simulink model "cx06_MA"  (Simulink 7.5)
settings: Solver=FixedStepDiscrete  StartTime=0.0  StopTime=10.0  RelTol=1e-3
undefined symbols (not defined in the file or in its folder): DiscIntNeverNeededParam, ECU555, int, motohawk_build_version, motohawk_trunc_name, motohawk_vardec_path
libraries: MotoHawk_lib x811, simulink x43, simulink_need_slupdate x1
(part 5 of 10)

== system cx06_MA/Strategy/A/C Control Code ==
  In1 : Inport  OutDataType=sfix(16)  OutScaling=2^0
  A/C StateMachine : Stateflow chart  TreatAsAtomicUnit=on
  Bus Creator : BusCreator  Inputs=1
  Bus Selector : BusSelector  OutputSignals="GMLAN.AC_Clutch_Req,Analog.AC_Pres,Fiat.Engine  General Status.Eng_Running_Stat"
  Constant : Constant  OutDataType=sfix(16)  OutScaling=2^0
  Constant1 : Constant  Value=0  OutDataType=sfix(16)  OutScaling=2^0
  Logical Operator : Logic  Inputs=5  AllPortsSameDT=off  OutDataTypeMode=boolean  OutDataTypeStr=boolean
  Logical Operator1 : Logic  Operator=NOT  AllPortsSameDT=off  OutDataTypeMode=boolean  OutDataTypeStr=boolean
  Relational Operator : RelationalOperator  Operator===  LogicOutDataTypeMode=boolean  OutDataTypeStr=boolean
  Relational Operator1 : RelationalOperator  Operator=>  LogicOutDataTypeMode=boolean  OutDataTypeStr=boolean
  motohawk_calibration2 : MotoHawk_lib/Calibration & Probing Blocks/motohawk_calibration  nam='off_Pres'  val=10  storage=Calibration  show_more=on  name_source=Use Parameter  data_type=double  read_level=1  write_level=1  ovr_cals=on  view_as=Number  enum_struct={'False', 'True'}  vector_style=Wide Row  use_help_units=off  help=''  units=''  use_header_enum=off  row_header_enum={}  col_header_enum={}  use_min_max=on  min_val=0  max_val=inf  use_precision=on  precision='1.2'  gain=1  offset=0  exp=1  use_mototune_group=off  mototune_group=motohawk_vardec_path(gcb)
  motohawk_calibration3 : MotoHawk_lib/Calibration & Probing Blocks/motohawk_calibration  nam='on_Pres'  val=10  storage=Calibration  show_more=on  name_source=Use Parameter  data_type=double  read_level=1  write_level=1  ovr_cals=on  view_as=Number  enum_struct={'False', 'True'}  vector_style=Wide Row  use_help_units=off  help=''  units=''  use_header_enum=off  row_header_enum={}  col_header_enum={}  use_min_max=on  min_val=0  max_val=inf  use_precision=on  precision='1.2'  gain=1  offset=0  exp=1  use_mototune_group=off  mototune_group=motohawk_vardec_path(gcb)
  motohawk_calibration4 : MotoHawk_lib/Calibration & Probing Blocks/motohawk_calibration  nam='Enable_AC'  val=0  storage=Calibration  show_more=on  name_source=Use Parameter  data_type=uint16  read_level=1  write_level=1  ovr_cals=on  view_as=Enumeration  enum_struct={'False', 'True'}  vector_style=Wide Row  use_help_units=off  help=''  units=''  use_header_enum=off  row_header_enum={}  col_header_enum={}  use_min_max=on  min_val=-inf  max_val=inf  use_precision=on  precision=''  gain=1  offset=0  exp=1  use_mototune_group=off  mototune_group=motohawk_vardec_path(gcb)
  motohawk_fault_action : MotoHawk_lib/Fault Management Blocks/motohawk_fault_action  nam='inhibitAC'  output_status=on  eval_nam=inhibitAC
  motohawk_probe1 : MotoHawk_lib/Calibration & Probing Blocks/motohawk_probe  nam='HVAC_Req'  show_more=on  name_source=Use Parameter  read_level=1  view_as=Number  enum_struct={'Safety', 'Diesel', 'Regen', 'HEV', 'ZEV'}  vector_style=Wide Row  use_help_units=off  help=''  units=''  use_header_enum=off  row_header_enum={}  col_header_enum={}  use_precision=off  precision=''  gain=1  offset=0  exp=1  use_mototune_group=off  mototune_group=motohawk_vardec_path(gcb)
  motohawk_probe2 : MotoHawk_lib/Calibration & Probing Blocks/motohawk_probe  nam='AC_Pressure'  show_more=on  name_source=Use Parameter  read_level=1  view_as=Number  enum_struct={'Safety', 'Diesel', 'Regen', 'HEV', 'ZEV'}  vector_style=Wide Row  use_help_units=off  help=''  units=''  use_header_enum=off  row_header_enum={}  col_header_enum={}  use_precision=off  precision=''  gain=1  offset=0  exp=1  use_mototune_group=off  mototune_group=motohawk_vardec_path(gcb)
  motohawk_probe3 : MotoHawk_lib/Calibration & Probing Blocks/motohawk_probe  nam='Pres_In_Range'  show_more=on  name_source=Use Parameter  read_level=1  view_as=Number  enum_struct={'Safety', 'Diesel', 'Regen', 'HEV', 'ZEV'}  vector_style=Wide Row  use_help_units=off  help=''  units=''  use_header_enum=off  row_header_enum={}  col_header_enum={}  use_precision=off  precision=''  gain=1  offset=0  exp=1  use_mototune_group=off  mototune_group=motohawk_vardec_path(gcb)
  Out1 : Outport  OutDataType=sfix(16)  OutScaling=2^0
  wires:
  Bus Creator/1 -> Out1/1
  In1/1 -> Bus Selector/1
  Bus Selector/1 -> Relational Operator/2  "<AC_Clutch_Req>"
  Logical Operator/1 -> Bus Creator/1  "AC_On"
  Bus Selector/2 -> A/C StateMachine/1(Pressure), motohawk_probe2/1  "<AC_Pres>"
  motohawk_calibration2/1 -> A/C StateMachine/2(off_Pres)
  motohawk_calibration3/1 -> A/C StateMachine/3(on_Pres)
  A/C StateMachine/1(activate) -> motohawk_probe3/1, Logical Operator/5
  motohawk_calibration4/1 -> Logical Operator/1
  motohawk_fault_action/1 -> Logical Operator1/1
  Logical Operator1/1 -> Logical Operator/3
  Relational Operator/1 -> Logical Operator/2, motohawk_probe1/1
  Constant/1 -> Relational Operator/1
  Bus Selector/3 -> Relational Operator1/1  "<Eng_Running_Stat>"
  Constant1/1 -> Relational Operator1/2
  Relational Operator1/1 -> Logical Operator/4

== system cx06_MA/Strategy/Fiat/GMLAN Control Code ==
  In1 : Inport  OutDataType=sfix(16)  OutScaling=2^0
  Bus Creator : BusCreator  Inputs=1
  Gear Calc : Subsystem
  Gear_Estimation : Subsystem
  Neutral Check : Subsystem
  motohawk_probe : MotoHawk_lib/Calibration & Probing Blocks/motohawk_probe  nam='Estimated_Gear'  show_more=on  name_source=Use Parameter  read_level=1  view_as=Number  enum_struct={'Disabled', 'Enabled'}  vector_style=Wide Row  use_help_units=off  help=''  units=''  use_header_enum=off  row_header_enum={}  col_header_enum={}  use_precision=off  precision=''  gain=1  offset=0  exp=1  use_mototune_group=off  mototune_group=motohawk_vardec_path(gcb)
  motohawk_probe1 : MotoHawk_lib/Calibration & Probing Blocks/motohawk_probe  nam='Exp_Neutral_Fault'  show_more=on  name_source=Use Parameter  read_level=1  view_as=Number  enum_struct={'Disabled', 'Enabled'}  vector_style=Wide Row  use_help_units=off  help=''  units=''  use_header_enum=off  row_header_enum={}  col_header_enum={}  use_precision=off  precision=''  gain=1  offset=0  exp=1  use_mototune_group=off  mototune_group=motohawk_vardec_path(gcb)
  Out1 : Outport  OutDataType=sfix(16)  OutScaling=2^0
  wires:
  In1/1 -> Gear Calc/1(In1), Gear_Estimation/1(In1), Neutral Check/2(In1)
  Gear Calc/1(gear) -> Bus Creator/1  "gear"
  Bus Creator/1 -> Out1/1
  Gear_Estimation/1(gear) -> Neutral Check/1(gear_In), Gear Calc/2(gear_In), motohawk_probe/1
  Neutral Check/1(fault) -> motohawk_probe1/1

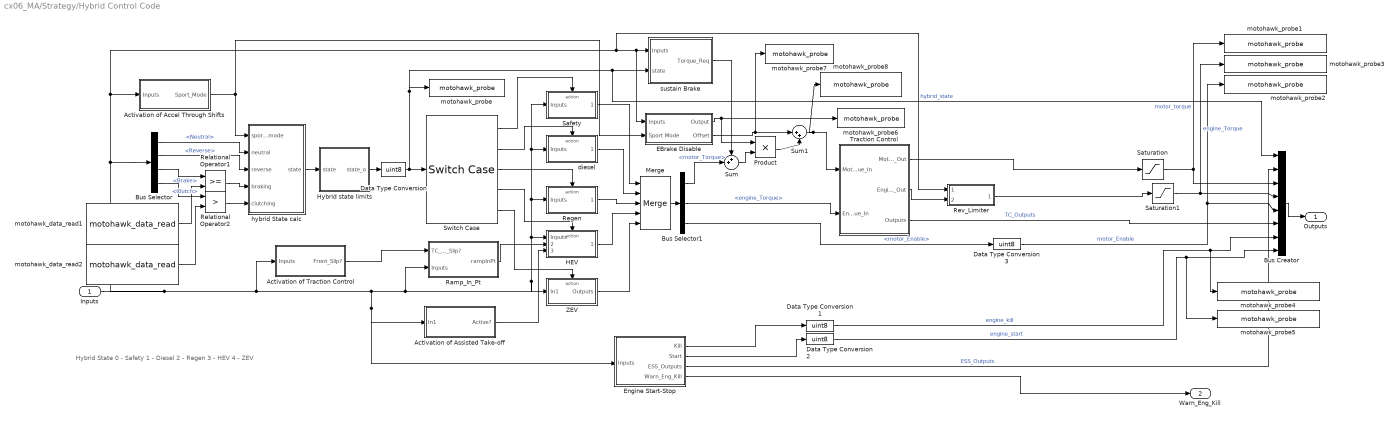
== system cx06_MA/Strategy/Hybrid Control Code ==
  note: Hybrid State
      | 0 - Safety
      | 1 - Diesel
      | 2 - Regen
      | 3 - HEV
      | 4 - ZEV
  Inputs : Inport  OutDataType=sfix(16)  OutScaling=2^0
  Activation of Accel Through Shifts : Subsystem
  Activation of Assisted Take-off : Subsystem
  Activation of Traction Control : Subsystem
  Bus Creator : BusCreator  Inputs=8
  Bus Selector : BusSelector  OutputSignals=Analog.Trans.Neutral,Analog.Trans.Reverse,Analog.Driver.Brake,Analog.Driver.Clutch
  Bus Selector1 : BusSelector  OutputSignals=motor_Torque,engine_Torque,motor_Enable
  Data Type Conversion{,1..3} (4 alike) : DataTypeConversion  OutDataTypeMode=uint8  OutDataType=sfix(16)  OutScaling=2^0  OutDataTypeStr=uint8
  EBrake Disable : Subsystem
  Engine Start-Stop : Subsystem
  HEV : Subsystem  TreatAsAtomicUnit=on
  Hybrid state limits : Subsystem
  Merge : Merge  Inputs=5
  Product : Product  OutDataType=sfix(16)  OutScaling=2^0  RndMeth=Zero
  Ramp_In_Pt : Subsystem
  Regen : Subsystem  TreatAsAtomicUnit=on
  Relational Operator1 : RelationalOperator  LogicOutDataTypeMode=boolean  OutDataTypeStr=boolean
  Relational Operator2 : RelationalOperator  Operator=>  LogicOutDataTypeMode=boolean  OutDataTypeStr=boolean
  Rev_Limiter : Subsystem
  Safety : Subsystem  TreatAsAtomicUnit=on
  Saturation : Saturate  UpperLimit=1  LowerLimit=-1
  Saturation1 : Saturate  UpperLimit=1  LowerLimit=0
  Sum : Sum  Inputs=++|  OutDataType=sfix(16)  OutScaling=2^0
  Sum1 : Sum  Inputs=|++  OutDataType=sfix(16)  OutScaling=2^0
  Switch Case : SwitchCase  CaseConditions={0,1,2,3,4}  ShowDefaultCase=off
  Traction Control : Subsystem
  ZEV : Subsystem  TreatAsAtomicUnit=on
  diesel : Subsystem  TreatAsAtomicUnit=on
  hybrid State calc : Stateflow chart  TreatAsAtomicUnit=on
  motohawk_data_read1 : MotoHawk_lib/Data Storage Blocks/motohawk_data_read  source=Lookup By Name  structure=Scalar  operation=Read scalar from location by index  sz_vec=4  sz_row=2  sz_col=3  typ=double  nam='Regen_Start'  checkNull=on  struct_inst_name='Struct1'  struct_nam='MyStruct'
  motohawk_data_read2 : MotoHawk_lib/Data Storage Blocks/motohawk_data_read  source=Lookup By Name  structure=Scalar  operation=Read scalar from location by index  sz_vec=4  sz_row=2  sz_col=3  typ=double  nam='AT_Start'  checkNull=on  struct_inst_name='Struct1'  struct_nam='MyStruct'
  motohawk_probe : MotoHawk_lib/Calibration & Probing Blocks/motohawk_probe  nam='Hybrid_State'  show_more=on  name_source=Use Parameter  read_level=1  view_as=Enumeration  enum_struct={'Safety', 'Diesel', 'Regen', 'HEV', 'ZEV'}  vector_style=Wide Row  use_help_units=off  help=''  units=''  use_header_enum=off  row_header_enum={}  col_header_enum={}  use_precision=off  precision=''  gain=1  offset=0  exp=1  use_mototune_group=off  mototune_group=motohawk_vardec_path(gcb)
  motohawk_probe1 : MotoHawk_lib/Calibration & Probing Blocks/motohawk_probe  nam='motor_Torque'  show_more=on  name_source=Use Parameter  read_level=1  view_as=Number  enum_struct={'Disabled', 'Enabled'}  vector_style=Wide Row  use_help_units=off  help=''  units=''  use_header_enum=off  row_header_enum={}  col_header_enum={}  use_precision=on  precision='1.3'  gain=1  offset=0  exp=1  use_mototune_group=off  mototune_group=motohawk_vardec_path(gcb)
  motohawk_probe2 : MotoHawk_lib/Calibration & Probing Blocks/motohawk_probe  nam='motor_Enable'  show_more=on  name_source=Use Parameter  read_level=1  view_as=Enumeration  enum_struct={'FALSE', 'true'}  vector_style=Wide Row  use_help_units=off  help=''  units=''  use_header_enum=off  row_header_enum={}  col_header_enum={}  use_precision=off  precision=''  gain=1  offset=0  exp=1  use_mototune_group=off  mototune_group=motohawk_vardec_path(gcb)
  motohawk_probe3 : MotoHawk_lib/Calibration & Probing Blocks/motohawk_probe  nam='diesel_Torque'  show_more=on  name_source=Use Parameter  read_level=1  view_as=Number  enum_struct={'Disabled', 'Enabled'}  vector_style=Wide Row  use_help_units=off  help=''  units=''  use_header_enum=off  row_header_enum={}  col_header_enum={}  use_precision=on  precision='1.3'  gain=1  offset=0  exp=1  use_mototune_group=off  mototune_group=motohawk_vardec_path(gcb)
  motohawk_probe4 : MotoHawk_lib/Calibration & Probing Blocks/motohawk_probe  nam='eng_Kill'  show_more=on  name_source=Use Parameter  read_level=1  view_as=Enumeration  enum_struct={'False', 'True'}  vector_style=Wide Row  use_help_units=off  help=''  units=''  use_header_enum=off  row_header_enum={}  col_header_enum={}  use_precision=on  precision=''  gain=1  offset=0  exp=1  use_mototune_group=off  mototune_group=motohawk_vardec_path(gcb)
  motohawk_probe5 : MotoHawk_lib/Calibration & Probing Blocks/motohawk_probe  nam='eng_Start'  show_more=on  name_source=Use Parameter  read_level=1  view_as=Enumeration  enum_struct={'False', 'True'}  vector_style=Wide Row  use_help_units=off  help=''  units=''  use_header_enum=off  row_header_enum={}  col_header_enum={}  use_precision=on  precision=''  gain=1  offset=0  exp=1  use_mototune_group=off  mototune_group=motohawk_vardec_path(gcb)
  motohawk_probe6 : MotoHawk_lib/Calibration & Probing Blocks/motohawk_probe  nam='EBrake_Multiplier'  show_more=on  name_source=Use Parameter  read_level=1  view_as=Number  enum_struct={'False', 'True'}  vector_style=Wide Row  use_help_units=off  help=''  units=''  use_header_enum=off  row_header_enum={}  col_header_enum={}  use_precision=on  precision='1.1'  gain=1  offset=0  exp=1  use_mototune_group=off  mototune_group=motohawk_vardec_path(gcb)
  motohawk_probe7 : MotoHawk_lib/Calibration & Probing Blocks/motohawk_probe  nam='EBrake_Offset'  show_more=on  name_source=Use Parameter  read_level=1  view_as=Number  enum_struct={'False', 'True'}  vector_style=Wide Row  use_help_units=off  help=''  units=''  use_header_enum=off  row_header_enum={}  col_header_enum={}  use_precision=on  precision='1.3'  gain=1  offset=0  exp=1  use_mototune_group=off  mototune_group=motohawk_vardec_path(gcb)
  motohawk_probe8 : MotoHawk_lib/Calibration & Probing Blocks/motohawk_probe  nam='Motor_Torque_Pre_Filt'  show_more=on  name_source=Use Parameter  read_level=1  view_as=Number  enum_struct={'False', 'True'}  vector_style=Wide Row  use_help_units=off  help=''  units=''  use_header_enum=off  row_header_enum={}  col_header_enum={}  use_precision=on  precision='1.3'  gain=1  offset=0  exp=1  use_mototune_group=off  mototune_group=motohawk_vardec_path(gcb)
  sustain Brake : Subsystem
  Outputs : Outport  OutDataType=sfix(16)  OutScaling=2^0
  Warn_Eng_Kill : Outport  Port=2  OutDataType=sfix(16)  OutScaling=2^0
  wires:
  Inputs/1 -> Bus Selector/1, Activation of Accel Through Shifts/1(Inputs), sustain Brake/1(Inputs), EBrake Disable/1(Inputs), Rev_Limiter/1(Inputs), ZEV/1(In1), HEV/1(Inputs), Safety/1(Inputs), diesel/1(Inputs), Regen/1(Inputs), Ramp_In_Pt/2(Inputs), Activation of Assisted Take-off/1(In1), Engine Start-Stop/1(Inputs), Activation of Traction Control/1(Inputs)
  Safety/1(Outputs) -> Merge/1
  diesel/1(Outputs) -> Merge/2
  HEV/1(Outputs) -> Merge/4
  ZEV/1(Outputs) -> Merge/5
  Regen/1(Outputs) -> Merge/3
  Switch Case/3 -> Regen/Action
  Switch Case/4 -> HEV/Action
  Switch Case/5 -> ZEV/Action
  Switch Case/2 -> diesel/Action
  Switch Case/1 -> Safety/Action
  Hybrid state limits/1(state_o) -> Data Type Conversion/1
  hybrid State calc/1(state) -> Hybrid state limits/1(state)
  Bus Selector/1 -> hybrid State calc/2(neutral)  "<Neutral>"
  Bus Selector/2 -> hybrid State calc/3(reverse)  "<Reverse>"
  Bus Selector/3 -> Relational Operator1/1  "<Brake>"
  Bus Selector/4 -> Relational Operator2/1  "<Clutch>"
  Relational Operator1/1 -> hybrid State calc/4(braking)
  Relational Operator2/1 -> hybrid State calc/5(clutching)
  motohawk_data_read1/1 -> Relational Operator1/2
  motohawk_data_read2/1 -> Relational Operator2/2
  Merge/1 -> Bus Selector1/1
  sustain Brake/1(Torque_Req) -> Sum/1
  Bus Selector1/1 -> Sum/2  "<motor_Torque>"
  Bus Creator/1 -> Outputs/1
  Data Type Conversion/1 -> Switch Case/1, motohawk_probe/1, sustain Brake/2("state "), Bus Creator/1  "hybrid_state"
  Data Type Conversion1/1 -> motohawk_probe4/1, Bus Creator/7  "engine_kill"
  Data Type Conversion2/1 -> motohawk_probe5/1, Bus Creator/8  "engine_start"
  Ramp_In_Pt/1(rampInPt) -> HEV/2(RampInPt)
  Traction Control/2(Engine_Torque_Out) -> Rev_Limiter/2(Torq_In)
  Saturation1/1 -> motohawk_probe3/1, Bus Creator/4  "engine_Torque"
  Saturation/1 -> motohawk_probe1/1, Bus Creator/3  "motor_torque"
  Bus Selector1/2 -> Traction Control/2(Engine_Torque_In)  "<engine_Torque>"
  Bus Selector1/3 -> Data Type Conversion3/1  "<motor_Enable>"
  Data Type Conversion3/1 -> motohawk_probe2/1, Bus Creator/5  "motor_Enable"
  Activation of Assisted Take-off/1(Active?) -> HEV/3(Activate_AT?)
  Activation of Traction Control/1(Front_Slip?) -> Ramp_In_Pt/1(TC_Front_Slip?)
  Activation of Accel Through Shifts/1(Sport_Mode) -> hybrid State calc/1(sport_mode), EBrake Disable/2(Sport Mode)
  Engine Start-Stop/3(ESS_Outputs) -> Bus Creator/2  "ESS_Outputs"
  Engine Start-Stop/1(Kill) -> Data Type Conversion1/1
  Engine Start-Stop/2(Start) -> Data Type Conversion2/1
  Traction Control/1(Motor_Torque_Out) -> Saturation/1
  Traction Control/3(Outputs) -> Bus Creator/6  "TC_Outputs"
  Rev_Limiter/1(Torq_Out) -> Saturation1/1
  EBrake Disable/1(Output) -> Product/1, motohawk_probe6/1
  Engine Start-Stop/4(Warn_Eng_Kill) -> Warn_Eng_Kill/1
  Sum/1 -> Product/2
  EBrake Disable/2(Offset) -> Sum1/1, motohawk_probe7/1
  Product/1 -> Sum1/2
  Sum1/1 -> Traction Control/1(Motor_Torque_In), motohawk_probe8/1

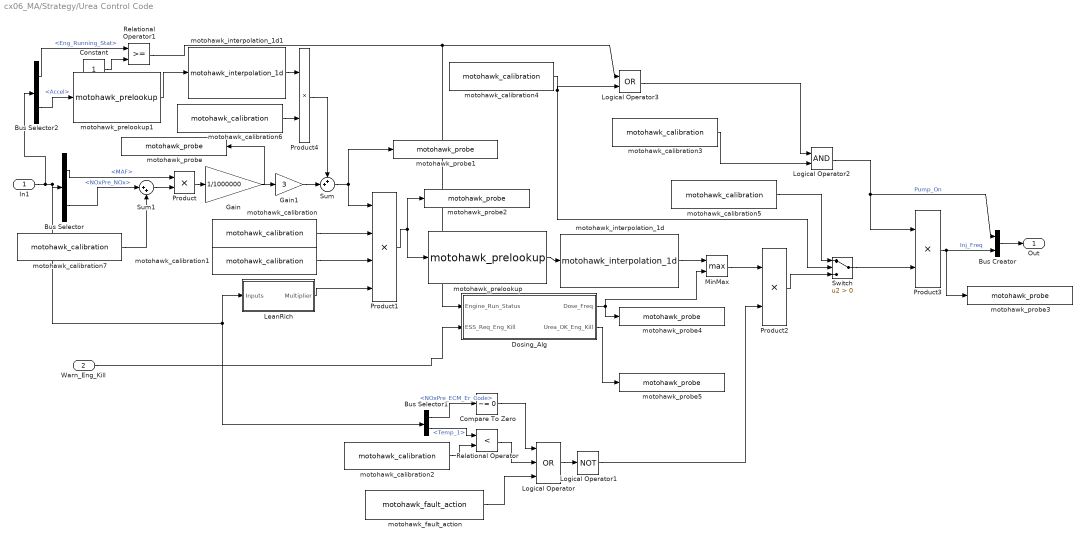
== system cx06_MA/Strategy/Urea Control Code ==
  In1 : Inport  OutDataType=sfix(16)  OutScaling=2^0
  Warn_Eng_Kill : Inport  Port=2  OutDataType=sfix(16)  OutScaling=2^0
  Bus Creator : BusCreator  Inputs=2
  Bus Selector : BusSelector  OutputSignals=Analog.MAF,Urea.NOx_Pre.NOxPre_NOx
  Bus Selector1 : BusSelector  OutputSignals=Urea.NOx_Pre.NOxPre_ECM_Er_Code,Urea.Temperature.Temp_1
  Bus Selector2 : BusSelector  OutputSignals="Fiat.Engine  General Status.Eng_Running_Stat,Analog.Driver.Accel"
  Compare To Zero : simulink/Logic and Bit Operations/Compare To Zero  SystemSampleTime=-1  relop=~=  LogicOutDataTypeMode=uint8  ZeroCross=off
  Constant : Constant  OutDataType=sfix(16)  OutScaling=2^0
  Dosing_Alg : Subsystem
  Gain : Gain  Gain=1/1000000  ParameterDataType=sfix(16)  ParameterScaling=2^0  OutDataType=sfix(16)  OutScaling=2^0
  Gain1 : Gain  Gain=3  ParameterDataType=sfix(16)  ParameterScaling=2^0  OutDataType=sfix(16)  OutScaling=2^0
  LeanRich : Subsystem
  Logical Operator : Logic  Operator=OR  Inputs=3  AllPortsSameDT=off  OutDataTypeMode=boolean  OutDataTypeStr=boolean
  Logical Operator1 : Logic  Operator=NOT  AllPortsSameDT=off  OutDataTypeMode=boolean  OutDataTypeStr=boolean
  Logical Operator2 : Logic  AllPortsSameDT=off  OutDataTypeMode=boolean  OutDataTypeStr=boolean
  Logical Operator3 : Logic  Operator=OR  AllPortsSameDT=off  OutDataTypeMode=boolean  OutDataTypeStr=boolean
  MinMax : MinMax  Function=max  Inputs=2  OutDataType=sfix(16)  OutScaling=2^0
  Product{,2..4} (4 alike) : Product  OutDataType=sfix(16)  OutScaling=2^0  RndMeth=Zero
  Product1 : Product  Inputs=4  OutDataType=sfix(16)  OutScaling=2^0  RndMeth=Zero
  Relational Operator : RelationalOperator  Operator=<  LogicOutDataTypeMode=boolean  OutDataTypeStr=boolean
  Relational Operator1 : RelationalOperator  LogicOutDataTypeMode=boolean  OutDataTypeStr=boolean
  Sum : Sum  Inputs=++|  OutDataType=sfix(16)  OutScaling=2^0
  Sum1 : Sum  Inputs=|++  OutDataType=sfix(16)  OutScaling=2^0
  Switch : Switch  Criteria=u2 > Threshold
  motohawk_calibration : MotoHawk_lib/Calibration & Probing Blocks/motohawk_calibration  nam='Urea_Dilution'  val=0  storage=Calibration  show_more=on  name_source=Use Parameter  data_type=Inherit from 'Default Value'  read_level=1  write_level=1  ovr_cals=on  view_as=Number  enum_struct={'Disabled', 'Enabled'}  vector_style=Wide Row  use_help_units=on  help='Dilution multiplier ureaMass * Urea_Dilution = SolutionMass'  units=''  use_header_enum=off  row_header_enum={}  col_header_enum={}  use_min_max=off  min_val=-inf  max_val=inf  use_precision=on  precision='1.3'  gain=1  offset=0  exp=1  use_mototune_group=off  mototune_group=motohawk_vardec_path(gcb)
  motohawk_calibration1 : MotoHawk_lib/Calibration & Probing Blocks/motohawk_calibration  nam='UreaNOx_Mult'  val=0  storage=Calibration  show_more=on  name_source=Use Parameter  data_type=Inherit from 'Default Value'  read_level=1  write_level=1  ovr_cals=on  view_as=Number  enum_struct={'Disabled', 'Enabled'}  vector_style=Wide Row  use_help_units=on  help='Multiplier to increase injection from NOx path'  units=''  use_header_enum=off  row_header_enum={}  col_header_enum={}  use_min_max=off  min_val=-inf  max_val=inf  use_precision=on  precision='1.3'  gain=1  offset=0  exp=1  use_mototune_group=off  mototune_group=motohawk_vardec_path(gcb)
  motohawk_calibration2 : MotoHawk_lib/Calibration & Probing Blocks/motohawk_calibration  nam='UreaMin_Temp'  val=0  storage=Calibration  show_more=on  name_source=Use Parameter  data_type=Inherit from 'Default Value'  read_level=1  write_level=1  ovr_cals=on  view_as=Number  enum_struct={'Disabled', 'Enabled'}  vector_style=Wide Row  use_help_units=on  help='Exhaust must be this hot to inject'  units=''  use_header_enum=off  row_header_enum={}  col_header_enum={}  use_min_max=off  min_val=-inf  max_val=inf  use_precision=on  precision='1.3'  gain=1  offset=0  exp=1  use_mototune_group=off  mototune_group=motohawk_vardec_path(gcb)
  motohawk_calibration3 : MotoHawk_lib/Calibration & Probing Blocks/motohawk_calibration  nam='Urea_Enable'  val=0  storage=Calibration  show_more=on  name_source=Use Parameter  data_type=boolean  read_level=1  write_level=1  ovr_cals=on  view_as=Enumeration  enum_struct={'Disabled', 'Enabled'}  vector_style=Wide Row  use_help_units=on  help=''  units=''  use_header_enum=off  row_header_enum={}  col_header_enum={}  use_min_max=off  min_val=-inf  max_val=inf  use_precision=on  precision='1.3'  gain=1  offset=0  exp=1  use_mototune_group=off  mototune_group=motohawk_vardec_path(gcb)
  motohawk_calibration4 : MotoHawk_lib/Calibration & Probing Blocks/motohawk_calibration  nam='Urea_Purge'  val=0  storage=Calibration  show_more=on  name_source=Use Parameter  data_type=boolean  read_level=1  write_level=1  ovr_cals=on  view_as=Enumeration  enum_struct={'Disabled', 'Enabled'}  vector_style=Wide Row  use_help_units=on  help='Set Injection to a fixed rate'  units=''  use_header_enum=off  row_header_enum={}  col_header_enum={}  use_min_max=off  min_val=-inf  max_val=inf  use_precision=on  precision='1.3'  gain=1  offset=0  exp=1  use_mototune_group=off  mototune_group=motohawk_vardec_path(gcb)
  motohawk_calibration5 : MotoHawk_lib/Calibration & Probing Blocks/motohawk_calibration  nam='Urea_PurgeLevel'  val=0  storage=Calibration  show_more=on  name_source=Use Parameter  data_type=Inherit from 'Default Value'  read_level=1  write_level=1  ovr_cals=on  view_as=Number  enum_struct={'Disabled', 'Enabled'}  vector_style=Wide Row  use_help_units=on  help=''  units='Hz'  use_header_enum=off  row_header_enum={}  col_header_enum={}  use_min_max=off  min_val=-inf  max_val=inf  use_precision=on  precision='1.1'  gain=1  offset=0  exp=1  use_mototune_group=off  mototune_group=motohawk_vardec_path(gcb)
  motohawk_calibration6 : MotoHawk_lib/Calibration & Probing Blocks/motohawk_calibration  nam='UreaAccel_Mult'  val=0  storage=Calibration  show_more=on  name_source=Use Parameter  data_type=Inherit from 'Default Value'  read_level=1  write_level=1  ovr_cals=on  view_as=Number  enum_struct={'Disabled', 'Enabled'}  vector_style=Wide Row  use_help_units=on  help='Multiplier to increase injection from NOx path'  units=''  use_header_enum=off  row_header_enum={}  col_header_enum={}  use_min_max=off  min_val=-inf  max_val=inf  use_precision=on  precision='1.3'  gain=1  offset=0  exp=1  use_mototune_group=off  mototune_group=motohawk_vardec_path(gcb)
  motohawk_calibration7 : MotoHawk_lib/Calibration & Probing Blocks/motohawk_calibration  nam='NOx_Offset'  val=0  storage=Calibration  show_more=on  name_source=Use Parameter  data_type=uint16  read_level=1  write_level=1  ovr_cals=on  view_as=Number  enum_struct={'Disabled', 'Enabled'}  vector_style=Wide Row  use_help_units=on  help='Dilution multiplier ureaMass * Urea_Dilution = SolutionMass'  units=''  use_header_enum=off  row_header_enum={}  col_header_enum={}  use_min_max=off  min_val=-inf  max_val=inf  use_precision=on  precision='1.1'  gain=1  offset=0  exp=1  use_mototune_group=off  mototune_group=motohawk_vardec_path(gcb)
  motohawk_fault_action : MotoHawk_lib/Fault Management Blocks/motohawk_fault_action  nam='Urea_Inject'  output_status=on  eval_nam=Urea_Inject
  motohawk_interpolation_1d : MotoHawk_lib/Lookup Tables/motohawk_interpolation_1d  nam='Urea_Injection_Tbl'  table_data=1:1:10  show_more=on  data_type=Inherit from 'Table Data'  storage=NonAdaptive  read_level=1  write_level=1  ovr_cals=on  use_help=off  help=''  units=''  use_min_max=off  min_val=-inf  max_val=inf  use_precision=off  precision=''  gain=1  offset=0  exp=1  use_links=on  prelookup_block='Urea_Injection_Ord'  output_name=''  use_mototune_group=off  mototune_group=motohawk_vardec_path(gcb)
  motohawk_interpolation_1d1 : MotoHawk_lib/Lookup Tables/motohawk_interpolation_1d  nam='Urea_Accel_Tbl'  table_data=1:1:10  show_more=on  data_type=Inherit from 'Table Data'  storage=NonAdaptive  read_level=1  write_level=1  ovr_cals=on  use_help=off  help=''  units=''  use_min_max=off  min_val=-inf  max_val=inf  use_precision=off  precision=''  gain=1  offset=0  exp=1  use_links=on  prelookup_block='Urea_Accel_Ord'  output_name=''  use_mototune_group=off  mototune_group=motohawk_vardec_path(gcb)
  motohawk_prelookup : MotoHawk_lib/Lookup Tables/motohawk_prelookup  nam='Urea_Injection_Ord'  breakpoint_data=1:1:10  show_more=off  data_type=Inherit from 'Table Data'  storage=Constant  read_level=1  write_level=1  ovr_cals=on  use_help=off  help=''  units=''  use_min_max=off  min_val=-inf  max_val=inf  use_precision=off  precision=''  gain=1  offset=0  exp=1  use_links=off  input_name=''  use_mototune_group=off  mototune_group=motohawk_vardec_path(gcb)
  motohawk_prelookup1 : MotoHawk_lib/Lookup Tables/motohawk_prelookup  nam='Urea_Accel_Ord'  breakpoint_data=1:1:10  show_more=off  data_type=Inherit from 'Table Data'  storage=Constant  read_level=1  write_level=1  ovr_cals=on  use_help=off  help=''  units=''  use_min_max=off  min_val=-inf  max_val=inf  use_precision=off  precision=''  gain=1  offset=0  exp=1  use_links=off  input_name=''  use_mototune_group=off  mototune_group=motohawk_vardec_path(gcb)
  motohawk_probe : MotoHawk_lib/Calibration & Probing Blocks/motohawk_probe  nam='NOx_MFlow_Theory'  show_more=on  name_source=Use Parameter  read_level=1  view_as=Number  enum_struct={'Disabled', 'Enabled'}  vector_style=Wide Row  use_help_units=off  help=''  units=''  use_header_enum=off  row_header_enum={}  col_header_enum={}  use_precision=on  precision='1.3'  gain=1  offset=0  exp=1  use_mototune_group=off  mototune_group=motohawk_vardec_path(gcb)
  motohawk_probe1 : MotoHawk_lib/Calibration & Probing Blocks/motohawk_probe  nam='Urea_MFlow'  show_more=on  name_source=Use Parameter  read_level=1  view_as=Number  enum_struct={'Disabled', 'Enabled'}  vector_style=Wide Row  use_help_units=off  help=''  units=''  use_header_enum=off  row_header_enum={}  col_header_enum={}  use_precision=on  precision='1.3'  gain=1  offset=0  exp=1  use_mototune_group=off  mototune_group=motohawk_vardec_path(gcb)
  motohawk_probe2 : MotoHawk_lib/Calibration & Probing Blocks/motohawk_probe  nam='Solution_MFlow'  show_more=on  name_source=Use Parameter  read_level=1  view_as=Number  enum_struct={'Disabled', 'Enabled'}  vector_style=Wide Row  use_help_units=off  help=''  units=''  use_header_enum=off  row_header_enum={}  col_header_enum={}  use_precision=on  precision='1.3'  gain=1  offset=0  exp=1  use_mototune_group=off  mototune_group=motohawk_vardec_path(gcb)
  motohawk_probe3 : MotoHawk_lib/Calibration & Probing Blocks/motohawk_probe  nam='UreaInj_Freq'  show_more=off  name_source=Use Parameter  read_level=1  view_as=Number  enum_struct={'Disabled', 'Enabled'}  vector_style=Wide Row  use_help_units=off  help=''  units=''  use_header_enum=off  row_header_enum={}  col_header_enum={}  use_precision=off  precision=''  gain=1  offset=0  exp=1  use_mototune_group=off  mototune_group=motohawk_vardec_path(gcb)
  motohawk_probe4 : MotoHawk_lib/Calibration & Probing Blocks/motohawk_probe  nam='Dosing_Freq'  show_more=on  name_source=Use Parameter  read_level=1  view_as=Number  enum_struct={'Disabled', 'Enabled'}  vector_style=Wide Row  use_help_units=off  help=''  units=''  use_header_enum=off  row_header_enum={}  col_header_enum={}  use_precision=on  precision='1.3'  gain=1  offset=0  exp=1  use_mototune_group=off  mototune_group=motohawk_vardec_path(gcb)
  motohawk_probe5 : MotoHawk_lib/Calibration & Probing Blocks/motohawk_probe  nam='Urea_OK_Eng_Kill'  show_more=on  name_source=Use Parameter  read_level=1  view_as=Number  enum_struct={'Disabled', 'Enabled'}  vector_style=Wide Row  use_help_units=off  help=''  units=''  use_header_enum=off  row_header_enum={}  col_header_enum={}  use_precision=on  precision='1.1'  gain=1  offset=0  exp=1  use_mototune_group=off  mototune_group=motohawk_vardec_path(gcb)
  Out : Outport  OutDataType=sfix(16)  OutScaling=2^0
  wires:
  In1/1 -> Bus Selector/1, Bus Selector1/1, LeanRich/1(Inputs), Bus Selector2/1
  Bus Selector/1 -> Product/1  "<MAF>"
  Product/1 -> Gain/1
  Gain/1 -> motohawk_probe/1, Gain1/1
  motohawk_calibration/1 -> Product1/2
  Product1/1 -> motohawk_probe2/1, motohawk_prelookup/1
  motohawk_calibration1/1 -> Product1/3
  motohawk_prelookup/1 -> motohawk_interpolation_1d/1
  Bus Selector1/2 -> Relational Operator/1  "<Temp_1>"
  motohawk_calibration2/1 -> Relational Operator/2
  Logical Operator/1 -> Logical Operator1/1
  Logical Operator1/1 -> Product2/2
  Product2/1 -> Switch/3
  motohawk_calibration4/1 -> Switch/2, Logical Operator3/2
  motohawk_calibration5/1 -> Switch/1
  Switch/1 -> Product3/2
  Product3/1 -> Bus Creator/2, motohawk_probe3/1  "Inj_Freq"
  Bus Creator/1 -> Out/1
  Bus Selector1/1 -> Compare To Zero/1  "<NOxPre_ECM_Er_Code>"
  Compare To Zero/1 -> Logical Operator/1
  Relational Operator/1 -> Logical Operator/2
  motohawk_fault_action/1 -> Logical Operator/3
  motohawk_prelookup1/1 -> motohawk_interpolation_1d1/1
  motohawk_interpolation_1d1/1 -> Product4/1
  motohawk_calibration6/1 -> Product4/2
  Product4/1 -> Sum/1
  Gain1/1 -> Sum/2
  Sum/1 -> Product1/1, motohawk_probe1/1
  LeanRich/1(Multiplier) -> Product1/4
  Bus Selector2/2 -> motohawk_prelookup1/1  "<Accel>"
  motohawk_calibration3/1 -> Logical Operator2/2
  Logical Operator2/1 -> Product3/1, Bus Creator/1  "Pump_On"
  Logical Operator3/1 -> Logical Operator2/1
  Bus Selector2/1 -> Relational Operator1/1  "<Eng_Running_Stat>"
  Relational Operator1/1 -> Logical Operator3/1, Dosing_Alg/1(Engine_Run_Status)
  Constant/1 -> Relational Operator1/2
  motohawk_interpolation_1d/1 -> MinMax/1
  Dosing_Alg/1(Dose_Freq) -> MinMax/2, motohawk_probe4/1
  MinMax/1 -> Product2/1
  Warn_Eng_Kill/1 -> Dosing_Alg/2(ESS_Req_Eng_Kill)
  Dosing_Alg/2(Urea_OK_Eng_Kill) -> motohawk_probe5/1
  Sum1/1 -> Product/2
  motohawk_calibration7/1 -> Sum1/2
  Bus Selector/2 -> Sum1/1  "<NOxPre_NOx>"

== system cx06_MA/Inputs/Analog Inputs/AC_Pres ==
  Compare To Zero : simulink/Logic and Bit Operations/Compare To Zero  SystemSampleTime=-1  relop=~=  LogicOutDataTypeMode=boolean  ZeroCross=off
  Relational Operator : RelationalOperator  Operator=<  LogicOutDataTypeMode=boolean  OutDataTypeStr=boolean
  motohawk_ain1 : MotoHawk_lib/Analog I//O Blocks/motohawk_ain  res_name=[]  text_resource=(None)  code_resource=NONE  val_resource=-1  target=ECU555-80  resource_enum_str=(None)=-1,ECUP=53,DRVP=54,XDRP=55,AN1M=56,AN2M=57,AN3M=58,AN4M=59,AN5M=60,AN6M=61,AN7M=62,AN8M=63,AN9M=64,AN10M=65,AN11M=66,AN12M=67,AN13M=68,AN14M=69,AN15M=70,AN16M=71,AN17M=72,AN18M=73,AN19M=74,O2A=90,O2B=91,XDRP_B=92  altref=5V Reference  typ=uint16  num_adc_bits=10  use_stat=on  use_vardec=on  nam='AC_Pres'  read_level=1  write_level=1  group='I/O Pins | Inputs Config'
  motohawk_calibration1 : MotoHawk_lib/Calibration & Probing Blocks/motohawk_calibration  nam='min_Press_Thres'  val=10  storage=Calibration  show_more=on  name_source=Use Parameter  data_type=uint16  read_level=1  write_level=1  ovr_cals=on  view_as=Number  enum_struct={'False', 'True'}  vector_style=Wide Row  use_help_units=off  help=''  units=''  use_header_enum=off  row_header_enum={}  col_header_enum={}  use_min_max=on  min_val=-inf  max_val=inf  use_precision=on  precision=''  gain=1  offset=0  exp=1  use_mototune_group=off  mototune_group=motohawk_vardec_path(gcb)
  motohawk_fault_def1 : MotoHawk_lib/Fault Management Blocks/motohawk_fault_def  nam='ACAnalogErr'  mode=Enabled - Persistent  id=[]  x=10  y=20  input_suspected=on  indeterminate=off  increment_xy=on  downsample_count=1  ovr_cals=on  ovr_actions=on  show_actions=on  action1_name='inhibitAC'  action1_cond=Active  action2_name=''  action2_cond=(None)  action3_name=''  action3_cond=(None)  action4_name=''  action4_cond=(None)
  motohawk_fault_def3 : MotoHawk_lib/Fault Management Blocks/motohawk_fault_def  nam='ACLowPres'  mode=Enabled - Persistent  id=[]  x=10  y=20  input_suspected=on  indeterminate=off  increment_xy=on  downsample_count=1  ovr_cals=on  ovr_actions=on  show_actions=on  action1_name='inhibitAC'  action1_cond=Active  action2_name=''  action2_cond=(None)  action3_name=''  action3_cond=(None)  action4_name=''  action4_cond=(None)
  motohawk_interpolation_1d : MotoHawk_lib/Lookup Tables/motohawk_interpolation_1d  nam='AC_Cal_Tbl'  table_data=[1:1:9]  show_more=off  data_type=Inherit from 'Table Data'  storage=NonAdaptive  read_level=1  write_level=1  ovr_cals=on  use_help=off  help=''  units=''  use_min_max=off  min_val=-inf  max_val=inf  use_precision=off  precision=''  gain=1  offset=0  exp=1  use_links=off  prelookup_block=''  output_name=''  use_mototune_group=off  mototune_group=motohawk_vardec_path(gcb)
  motohawk_prelookup : MotoHawk_lib/Lookup Tables/motohawk_prelookup  nam='AC_Cal_Ord'  breakpoint_data=[0:128:1024]  show_more=on  data_type=uint16  storage=Constant  read_level=1  write_level=1  ovr_cals=off  use_help=off  help=''  units=''  use_min_max=off  min_val=-inf  max_val=inf  use_precision=off  precision=''  gain=1  offset=0  exp=1  use_links=off  input_name=''  use_mototune_group=off  mototune_group=motohawk_vardec_path(gcb)
  motohawk_probe1 : MotoHawk_lib/Calibration & Probing Blocks/motohawk_probe  nam='In_ACPres'  show_more=on  name_source=Use Parameter  read_level=1  view_as=Number  enum_struct={'Disabled', 'Enabled'}  vector_style=Wide Row  use_help_units=off  help=''  units=''  use_header_enum=off  row_header_enum={}  col_header_enum={}  use_precision=off  precision=''  gain=1  offset=0  exp=1  use_mototune_group=on  mototune_group='Debug | Inputs'
  AC_Pres : Outport  OutDataType=sfix(16)  OutScaling=2^0
  wires:
  motohawk_ain1/1 -> motohawk_prelookup/1
  motohawk_prelookup/1 -> motohawk_interpolation_1d/1
  motohawk_interpolation_1d/1 -> AC_Pres/1, Relational Operator/1  "AC_Pres"
  motohawk_ain1/2 -> motohawk_probe1/1, Compare To Zero/1
  motohawk_calibration1/1 -> Relational Operator/2
  Relational Operator/1 -> motohawk_fault_def3/1
  Compare To Zero/1 -> motohawk_fault_def1/1

== system cx06_MA/Inputs/Analog Inputs/Cruise Buttons ==
  note: 0 - (none)
      | 1 - on
      | 2 - on & up
      | 3 - on & down
  motohawk_ain2 : MotoHawk_lib/Analog I//O Blocks/motohawk_ain  res_name=[]  text_resource=AN5M  code_resource=NONE  val_resource=-1  target=ECU555-80  resource_enum_str=(None)=-1,ECUP=53,DRVP=54,XDRP=55,AN1M=56,AN2M=57,AN3M=58,AN4M=59,AN5M=60,AN6M=61,AN7M=62,AN8M=63,AN9M=64,AN10M=65,AN11M=66,AN12M=67,AN13M=68,AN14M=69,AN15M=70,AN16M=71,AN17M=72,AN18M=73,AN19M=74,O2A=90,O2B=91,XDRP_B=92  altref=5V Reference  typ=uint16  num_adc_bits=10  use_stat=on  use_vardec=on  nam='CruiseButtons'  read_level=1  write_level=1  group='I/O Pins | Inputs Config'
  motohawk_calibration1 : MotoHawk_lib/Calibration & Probing Blocks/motohawk_calibration  nam='Cruise_Main_Tres'  val=50  storage=Calibration  show_more=on  name_source=Use Parameter  data_type=Inherit via back propagation  read_level=1  write_level=1  ovr_cals=on  view_as=Number  enum_struct={'Disabled', 'Enabled'}  vector_style=Wide Row  use_help_units=off  help=''  units=''  use_header_enum=off  row_header_enum={}  col_header_enum={}  use_min_max=on  min_val=0  max_val=inf  use_precision=off  precision=''  gain=1  offset=0  exp=1  use_mototune_group=off  mototune_group=motohawk_vardec_path(gcb)
  motohawk_calibration2 : MotoHawk_lib/Calibration & Probing Blocks/motohawk_calibration  nam='Cruise_Up_Tres'  val=50  storage=Calibration  show_more=on  name_source=Use Parameter  data_type=Inherit via back propagation  read_level=1  write_level=1  ovr_cals=on  view_as=Number  enum_struct={'Disabled', 'Enabled'}  vector_style=Wide Row  use_help_units=off  help=''  units=''  use_header_enum=off  row_header_enum={}  col_header_enum={}  use_min_max=on  min_val=0  max_val=inf  use_precision=off  precision=''  gain=1  offset=0  exp=1  use_mototune_group=off  mototune_group=motohawk_vardec_path(gcb)
  motohawk_calibration3 : MotoHawk_lib/Calibration & Probing Blocks/motohawk_calibration  nam='Cruise_Down_Tres'  val=50  storage=Calibration  show_more=on  name_source=Use Parameter  data_type=Inherit via back propagation  read_level=1  write_level=1  ovr_cals=on  view_as=Number  enum_struct={'Disabled', 'Enabled'}  vector_style=Wide Row  use_help_units=off  help=''  units=''  use_header_enum=off  row_header_enum={}  col_header_enum={}  use_min_max=on  min_val=0  max_val=inf  use_precision=off  precision=''  gain=1  offset=0  exp=1  use_mototune_group=off  mototune_group=motohawk_vardec_path(gcb)
  motohawk_probe6 : MotoHawk_lib/Calibration & Probing Blocks/motohawk_probe  nam='In_CruiseButtons'  show_more=on  name_source=Use Parameter  read_level=1  view_as=Number  enum_struct={'Disabled', 'Enabled'}  vector_style=Wide Row  use_help_units=off  help=''  units=''  use_header_enum=off  row_header_enum={}  col_header_enum={}  use_precision=off  precision=''  gain=1  offset=0  exp=1  use_mototune_group=on  mototune_group='Debug | Inputs'
  motohawk_probe9 : MotoHawk_lib/Calibration & Probing Blocks/motohawk_probe  nam='raw_CruiseButton'  show_more=on  name_source=Use Parameter  read_level=1  view_as=Number  enum_struct={'Disabled', 'Enabled'}  vector_style=Wide Row  use_help_units=on  help=''  units=''  use_header_enum=off  row_header_enum={}  col_header_enum={}  use_precision=off  precision=''  gain=1  offset=0  exp=1  use_mototune_group=off  mototune_group=motohawk_vardec_path(gcb)
  read_Cruise_Buttons : Stateflow chart  TreatAsAtomicUnit=on
  Cruise_Button : Outport  OutDataType=sfix(16)  OutScaling=2^0
  wires:
  motohawk_ain2/2 -> motohawk_probe6/1
  motohawk_ain2/1 -> motohawk_probe9/1, read_Cruise_Buttons/1(u)
  motohawk_calibration1/1 -> read_Cruise_Buttons/2(b1)
  motohawk_calibration2/1 -> read_Cruise_Buttons/3(b2)
  motohawk_calibration3/1 -> read_Cruise_Buttons/4(b3)
  read_Cruise_Buttons/1(cruiseBut) -> Cruise_Button/1  "cruiseBut"

== system cx06_MA/Inputs/Analog Inputs/Driver Inputs ==
  Accel : Subsystem
  Brake : Subsystem
  Bus Creator : BusCreator  Inputs=3
  Clutch : Subsystem
  Driver : Outport  OutDataType=sfix(16)  OutScaling=2^0
  wires:
  Bus Creator/1 -> Driver/1
  Accel/1(Accel) -> Bus Creator/1  "Accel"
  Brake/1(Brake) -> Bus Creator/2  "Brake"
  Clutch/1(Clutch) -> Bus Creator/3  "Clutch"

== system cx06_MA/Inputs/Analog Inputs/Fuel Level ==
  2pt Calibration1_4 : Fcn  Expr=(u[1]-u[3])/(u[2]-u[3])
  Data Type Conversion3 : DataTypeConversion  OutDataTypeMode=single  OutDataType=sfix(16)  OutScaling=2^0  OutDataTypeStr=single
  Mux4 : Mux  Inputs=3
  Range_Detect : Subsystem
  Saturation3 : Saturate  UpperLimit=1  LowerLimit=0
  motohawk_ain3 : MotoHawk_lib/Analog I//O Blocks/motohawk_ain  res_name=[]  text_resource=AN13M  code_resource=NONE  val_resource=-1  target=ECU555-80  resource_enum_str=(None)=-1,ECUP=53,DRVP=54,XDRP=55,AN1M=56,AN2M=57,AN3M=58,AN4M=59,AN5M=60,AN6M=61,AN7M=62,AN8M=63,AN9M=64,AN10M=65,AN11M=66,AN12M=67,AN13M=68,AN14M=69,AN15M=70,AN16M=71,AN17M=72,AN18M=73,AN19M=74,O2A=90,O2B=91,XDRP_B=92  altref=5V Reference  typ=uint16  num_adc_bits=10  use_stat=on  use_vardec=on  nam='FuelLevel'  read_level=1  write_level=1  group='I/O Pins | Inputs Config'
  motohawk_calibration7 : MotoHawk_lib/Calibration & Probing Blocks/motohawk_calibration  nam='FeulLevel_Zero'  val=416  storage=Calibration  show_more=on  name_source=Use Parameter  data_type=Inherit via back propagation  read_level=1  write_level=1  ovr_cals=on  view_as=Number  enum_struct={'Disabled', 'Enabled'}  vector_style=Wide Row  use_help_units=off  help=''  units=''  use_header_enum=off  row_header_enum={}  col_header_enum={}  use_min_max=off  min_val=-inf  max_val=inf  use_precision=off  precision=''  gain=1  offset=0  exp=1  use_mototune_group=off  mototune_group=motohawk_vardec_path(gcb)
  motohawk_calibration8 : MotoHawk_lib/Calibration & Probing Blocks/motohawk_calibration  nam='FuelLevel_Full'  val=231  storage=Calibration  show_more=on  name_source=Use Parameter  data_type=Inherit via back propagation  read_level=1  write_level=1  ovr_cals=on  view_as=Number  enum_struct={'Disabled', 'Enabled'}  vector_style=Wide Row  use_help_units=off  help=''  units=''  use_header_enum=off  row_header_enum={}  col_header_enum={}  use_min_max=off  min_val=-inf  max_val=inf  use_precision=off  precision=''  gain=1  offset=0  exp=1  use_mototune_group=off  mototune_group=motohawk_vardec_path(gcb)
  motohawk_fault_def : MotoHawk_lib/Fault Management Blocks/motohawk_fault_def  nam='FuelLevelRange'  mode=Disabled  id=[]  x=10  y=20  input_suspected=on  indeterminate=off  increment_xy=on  downsample_count=1  ovr_cals=on  ovr_actions=on  show_actions=off  action1_name=''  action1_cond=(None)  action2_name=''  action2_cond=(None)  action3_name=''  action3_cond=(None)  action4_name=''  action4_cond=(None)
  motohawk_probe3 : MotoHawk_lib/Calibration & Probing Blocks/motohawk_probe  nam='In_FuelLevel'  show_more=on  name_source=Use Parameter  read_level=1  view_as=Number  enum_struct={'Disabled', 'Enabled'}  vector_style=Wide Row  use_help_units=off  help=''  units=''  use_header_enum=off  row_header_enum={}  col_header_enum={}  use_precision=off  precision=''  gain=1  offset=0  exp=1  use_mototune_group=on  mototune_group='Debug | Inputs'
  motohawk_probe7 : MotoHawk_lib/Calibration & Probing Blocks/motohawk_probe  nam='raw_FuelLevel'  show_more=on  name_source=Use Parameter  read_level=1  view_as=Number  enum_struct={'Disabled', 'Enabled'}  vector_style=Wide Row  use_help_units=on  help=''  units=''  use_header_enum=off  row_header_enum={}  col_header_enum={}  use_precision=off  precision=''  gain=1  offset=0  exp=1  use_mototune_group=off  mototune_group=motohawk_vardec_path(gcb)
  motohawk_probe8 : MotoHawk_lib/Calibration & Probing Blocks/motohawk_probe  nam='cal_FuelLevel'  show_more=on  name_source=Use Parameter  read_level=1  view_as=Number  enum_struct={'Disabled', 'Enabled'}  vector_style=Wide Row  use_help_units=off  help=''  units=''  use_header_enum=off  row_header_enum={}  col_header_enum={}  use_precision=off  precision=''  gain=1  offset=0  exp=1  use_mototune_group=off  mototune_group=motohawk_vardec_path(gcb)
  Fuel_Level : Outport  OutDataType=sfix(16)  OutScaling=2^0
  wires:
  motohawk_ain3/1 -> Data Type Conversion3/1, motohawk_probe7/1
  motohawk_calibration7/1 -> Mux4/2, Range_Detect/2(Zero)
  motohawk_calibration8/1 -> Mux4/3, Range_Detect/3(Full)
  Mux4/1 -> 2pt Calibration1_4/1
  2pt Calibration1_4/1 -> Saturation3/1
  Data Type Conversion3/1 -> Mux4/1, Range_Detect/1(Value)
  Saturation3/1 -> motohawk_probe8/1, Fuel_Level/1  "Fuel_Level"
  Range_Detect/1(Fault) -> motohawk_fault_def/1
  motohawk_ain3/2 -> motohawk_probe3/1

== system cx06_MA/Inputs/Analog Inputs/MAF ==
  Weighted Moving Average : simulink_need_slupdate/Weighted Moving Average  mgainval=ones(1,25)./25  vinit=0.0  samptime=-1  OutDataTypeStr=Inherit: Inherit via back propagation  OutDataType=sfix(16)  OutScaling=2^-10  DoSatur=off  GainDataType=sfix( 16 )  MatRadixGroup=Best Precision: Matrix-wise  GainScaling=2^-10
  motohawk_frequency_in : MotoHawk_lib/Advanced Digital I//O/motohawk_frequency_in  res_name=[]  text_resource=DG4M  code_resource=RES_DG1M  val_resource=-1  target=ECU555-80  resource_enum_str=(None)=-1,DG1M=93,DG2M=94,DG4M=96,CNK=100  ipwm=No Duty Cycle Measurement  itrig=off  Nmax=8  edge=Rising Edge  alias=Enabled  min_freq=10  sig=Digital Input  use_vardec=on  nam='MAF_Input'  read_level=1  write_level=1  group='I/O Pins | Inputs Config'  cal_group='I/O Pins | Frequency In Config'
  motohawk_interpolation_1d1 : MotoHawk_lib/Lookup Tables/motohawk_interpolation_1d  nam='MAF_Cal_Tbl'  table_data=1:1:17  show_more=on  data_type=Inherit from 'Table Data'  storage=NonAdaptive  read_level=1  write_level=1  ovr_cals=on  use_help=off  help=''  units=''  use_min_max=off  min_val=-inf  max_val=inf  use_precision=off  precision=''  gain=1  offset=0  exp=1  use_links=on  prelookup_block='MAF_Cal_Ord'  output_name=''  use_mototune_group=off  mototune_group=motohawk_vardec_path(gcb)
  motohawk_prelookup1 : MotoHawk_lib/Lookup Tables/motohawk_prelookup  nam='MAF_Cal_Ord'  breakpoint_data=1:1:17  show_more=on  data_type=Inherit from 'Table Data'  storage=NonVolatile  read_level=1  write_level=1  ovr_cals=on  use_help=off  help=''  units=''  use_min_max=off  min_val=-inf  max_val=inf  use_precision=on  precision=''  gain=0.01  offset=0  exp=1  use_links=off  input_name=''  use_mototune_group=off  mototune_group=motohawk_vardec_path(gcb)
  motohawk_probe2 : MotoHawk_lib/Calibration & Probing Blocks/motohawk_probe  nam='raw_filtMAF'  show_more=on  name_source=Use Parameter  read_level=1  view_as=Number  enum_struct={'Disabled', 'Enabled'}  vector_style=Wide Row  use_help_units=on  help=''  units=''  use_header_enum=off  row_header_enum={}  col_header_enum={}  use_precision=on  precision=''  gain=0.01  offset=0  exp=1  use_mototune_group=off  mototune_group=motohawk_vardec_path(gcb)
  motohawk_probe4 : MotoHawk_lib/Calibration & Probing Blocks/motohawk_probe  nam='cal_MAF'  show_more=on  name_source=Use Parameter  read_level=1  view_as=Number  enum_struct={'Disabled', 'Enabled'}  vector_style=Wide Row  use_help_units=off  help=''  units=''  use_header_enum=off  row_header_enum={}  col_header_enum={}  use_precision=off  precision=''  gain=1  offset=0  exp=1  use_mototune_group=off  mototune_group=motohawk_vardec_path(gcb)
  motohawk_probe5 : MotoHawk_lib/Calibration & Probing Blocks/motohawk_probe  nam='raw_MAF'  show_more=on  name_source=Use Parameter  read_level=1  view_as=Number  enum_struct={'Disabled', 'Enabled'}  vector_style=Wide Row  use_help_units=on  help=''  units=''  use_header_enum=off  row_header_enum={}  col_header_enum={}  use_precision=on  precision=''  gain=0.01  offset=0  exp=1  use_mototune_group=off  mototune_group=motohawk_vardec_path(gcb)
  MAF : Outport  OutDataType=sfix(16)  OutScaling=2^0
  wires:
  motohawk_prelookup1/1 -> motohawk_interpolation_1d1/1
  motohawk_frequency_in/1 -> Weighted Moving Average/1, motohawk_probe5/1
  Weighted Moving Average/1 -> motohawk_prelookup1/1, motohawk_probe2/1
  motohawk_interpolation_1d1/1 -> motohawk_probe4/1, MAF/1  "MAF"
